simulink model "clutch_lockup"  (R2020a)
settings: Solver=VariableStepAuto  StartTime=0.0  StopTime=10.0  RelTol=1e-3
undefined symbols (not defined in the file or in its folder): be, bv, Ie, Iv, muk, mus, R
settings Model: Creator=Shubham  LastModifiedBy=Shubham

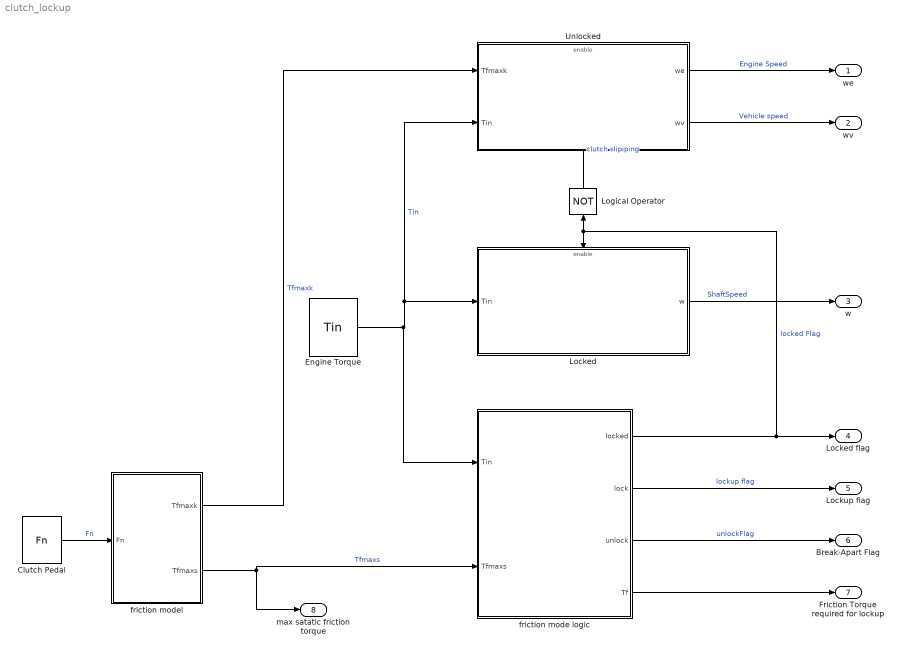
== system clutch_lockup ==
  Clutch Pedal : FromWorkspace  VariableName=Fn  ZeroCross=off
  Engine Torque : FromWorkspace  VariableName=Tin  ZeroCross=off
  Locked : Subsystem
  Logical Operator : Logic  Operator=NOT  IconShape=distinctive  AllPortsSameDT=off  OutDataTypeStr=boolean
  Unlocked : Subsystem
  friction mode logic : Subsystem  TreatAsAtomicUnit=on
  friction model : Subsystem
  we : Outport
  wv : Outport  Port=2
  w : Outport  Port=3
  Locked flag : Outport  Port=4
  Lockup flag : Outport  Port=5
  Break-Apart Flag : Outport  Port=6
  Friction Torque required for lockup : Outport  Port=7
  max satatic friction torque : Outport  Port=8
  wires:
  Engine Torque/1 -> friction mode logic/1(Tin), Locked/1(Tin), Unlocked/2(Tin)  "Tin"
  friction model/1(Tfmaxk) -> Unlocked/1(Tfmaxk)  "Tfmaxk"
  friction model/2(Tfmaxs) -> max satatic friction torque/1, friction mode logic/2(Tfmaxs)  "Tfmaxs"
  Clutch Pedal/1 -> friction model/1(Fn)  "Fn"
  Logical Operator/1 -> Unlocked/Enable  "clutch slipiping"
  Unlocked/1(we) -> we/1  "Engine Speed"
  Unlocked/2(wv) -> wv/1  "Vehicle speed"
  Locked/1(w) -> w/1  "ShaftSpeed"
  friction mode logic/2(lock) -> Lockup flag/1  "lockup flag"
  friction mode logic/3(unlock) -> Break-Apart Flag/1  "unlockFlag"
  friction mode logic/4(Tf) -> Friction Torque required for lockup/1
  friction mode logic/1(locked) -> Logical Operator/1, Locked/Enable, Locked flag/1  "locked Flag"

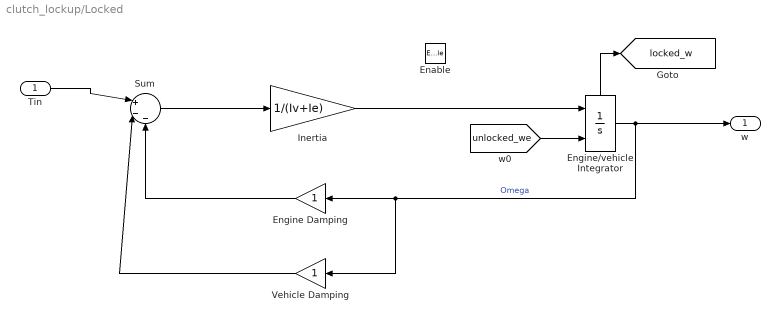
== system clutch_lockup/Locked ==
  Tin : Inport
  Enable : EnablePort  StatesWhenEnabling=reset
  Engine Damping : Gain
  Engine/vehicle Integrator : Integrator  InitialConditionSource=external  ShowStatePort=on
  Inertia : Gain  Gain=1/(Iv+Ie)
  Sum : Sum  Inputs=|+--
  Vehicle Damping : Gain
  w : Outport
  tag scope: locked_w=global
  wires:
  Sum/1 -> Inertia/1
  Inertia/1 -> Engine/vehicle Integrator/1
  Tin/1 -> Sum/1
  Engine/vehicle Integrator/State -> [locked_w]
  [unlocked_we] -> Engine/vehicle Integrator/2
  Engine Damping/1 -> Sum/3
  Vehicle Damping/1 -> Sum/2
  Engine/vehicle Integrator/1 -> w/1, Vehicle Damping/1, Engine Damping/1  "Omega"

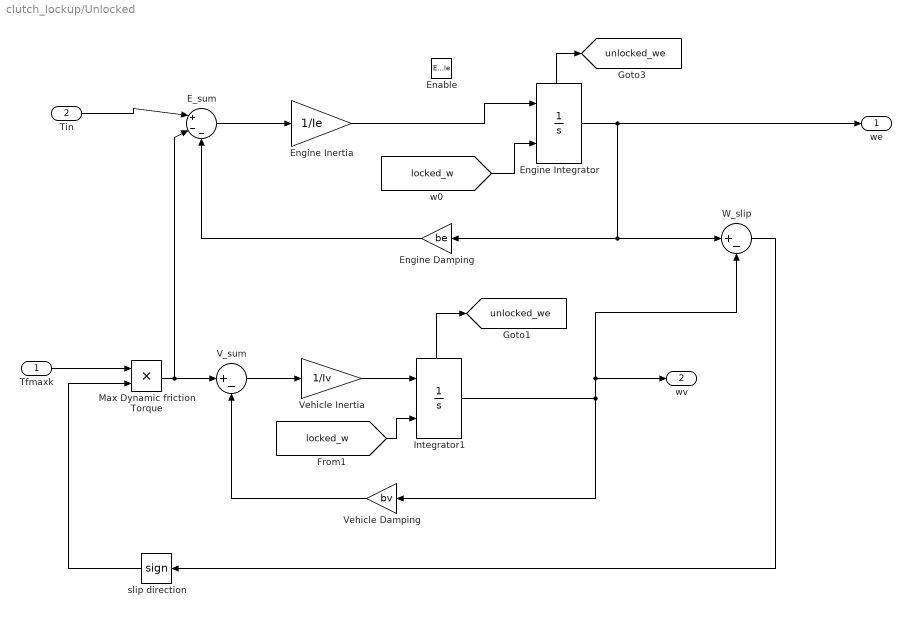
== system clutch_lockup/Unlocked ==
  Tfmaxk : Inport
  Tin : Inport  Port=2
  Enable : EnablePort  StatesWhenEnabling=reset
  E_sum : Sum  Inputs=|+--
  Engine Damping : Gain  Gain=be
  Engine Inertia : Gain  Gain=1/Ie
  Engine Integrator : Integrator  InitialConditionSource=external  ShowStatePort=on
  Integrator1 : Integrator  InitialConditionSource=external  ShowStatePort=on
  Max Dynamic friction Torque : Product
  V_sum : Sum  Inputs=|+-
  Vehicle Damping : Gain  Gain=bv
  Vehicle Inertia : Gain  Gain=1/Iv
  W_slip : Sum  Inputs=|+-
  slip direction : Signum
  we : Outport
  wv : Outport  Port=2
  tag scope: unlocked_we=global
  wires:
  Tin/1 -> E_sum/1
  E_sum/1 -> Engine Inertia/1
  Engine Inertia/1 -> Engine Integrator/1
  Engine Integrator/1 -> W_slip/1, Engine Damping/1, we/1
  Engine Damping/1 -> E_sum/3
  Vehicle Inertia/1 -> Integrator1/1
  V_sum/1 -> Vehicle Inertia/1
  Integrator1/1 -> W_slip/2, wv/1, Vehicle Damping/1
  Vehicle Damping/1 -> V_sum/2
  W_slip/1 -> slip direction/1
  slip direction/1 -> Max Dynamic friction Torque/2
  Max Dynamic friction Torque/1 -> E_sum/2, V_sum/1
  Tfmaxk/1 -> Max Dynamic friction Torque/1
  Engine Integrator/State -> [unlocked_we]
  Integrator1/State -> [unlocked_we]
  [locked_w] -> Engine Integrator/2
  [locked_w] -> Integrator1/2

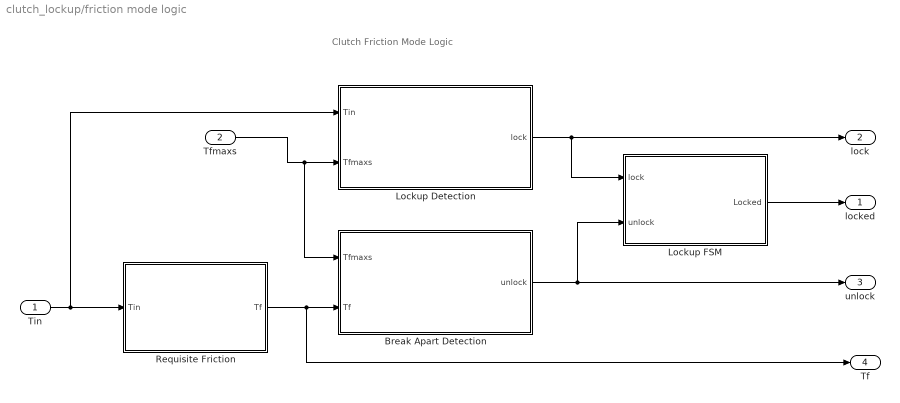
== system clutch_lockup/friction mode logic ==
  note: Clutch Friction Mode Logic
  Tin : Inport
  Tfmaxs : Inport  Port=2
  "Break Apart Detection " : Subsystem
  Lockup Detection : Subsystem
  Lockup FSM : Subsystem
  "Requisite Friction " : Subsystem
  locked : Outport
  lock : Outport  Port=2
  unlock : Outport  Port=3
  Tf : Outport  Port=4
  wires:
  "Requisite Friction "/1(Tf) -> "Break Apart Detection "/2(Tf), Tf/1
  Tin/1 -> "Requisite Friction "/1(Tin), Lockup Detection/1(Tin)
  Tfmaxs/1 -> "Break Apart Detection "/1(Tfmaxs), Lockup Detection/2(Tfmaxs)
  Lockup Detection/1(lock) -> Lockup FSM/1(lock), lock/1
  Lockup FSM/1(Locked) -> locked/1
  "Break Apart Detection "/1(unlock) -> Lockup FSM/2(unlock), unlock/1

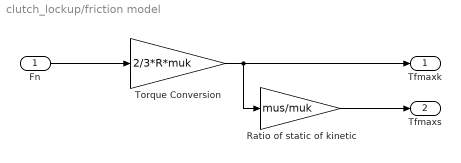
== system clutch_lockup/friction model ==
  Fn : Inport
  Ratio of static of kinetic : Gain  Gain=mus/muk
  Torque Conversion : Gain  Gain=2/3*R*muk
  Tfmaxk : Outport
  Tfmaxs : Outport  Port=2
  wires:
  Fn/1 -> Torque Conversion/1
  Torque Conversion/1 -> Tfmaxk/1, Ratio of static of kinetic/1
  Ratio of static of kinetic/1 -> Tfmaxs/1

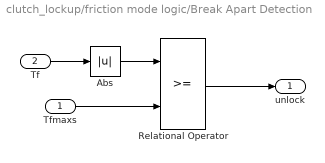
== system clutch_lockup/friction mode logic/Break Apart Detection  ==
  Tfmaxs : Inport
  Tf : Inport  Port=2
  Abs : Abs
  Relational Operator : RelationalOperator  OutDataTypeStr=boolean  RndMeth=Simplest
  unlock : Outport
  wires:
  Tf/1 -> Abs/1
  Relational Operator/1 -> unlock/1
  Abs/1 -> Relational Operator/1
  Tfmaxs/1 -> Relational Operator/2

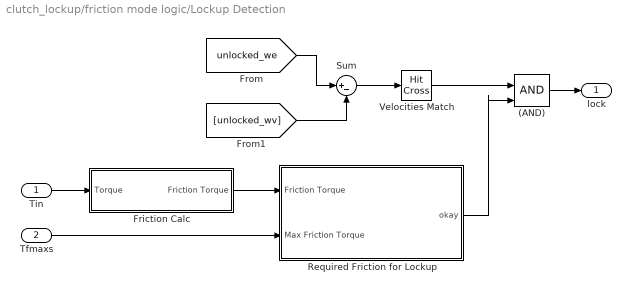
== system clutch_lockup/friction mode logic/Lockup Detection ==
  Tin : Inport
  Tfmaxs : Inport  Port=2
  (AND) : Logic  IconShape=distinctive  AllPortsSameDT=off  OutDataTypeStr=boolean
  Friction Calc : Subsystem
  Required Friction for Lockup : Subsystem
  Sum : Sum  Inputs=|+-
  Velocities Match : HitCross
  lock : Outport
  wires:
  Required Friction for Lockup/1(okay) -> (AND)/2
  (AND)/1 -> lock/1
  Tin/1 -> Friction Calc/1(Torque)
  Friction Calc/1(Friction Torque) -> Required Friction for Lockup/1(Friction Torque)
  Tfmaxs/1 -> Required Friction for Lockup/2(Max Friction Torque)
  Velocities Match/1 -> (AND)/1
  Sum/1 -> Velocities Match/1
  [unlocked_wv] -> Sum/2
  [unlocked_we] -> Sum/1

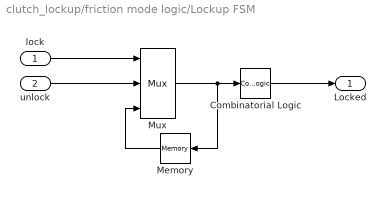
== system clutch_lockup/friction mode logic/Lockup FSM ==
  lock : Inport
  unlock : Inport  Port=2
  Combinatorial Logic : CombinatorialLogic  TruthTable=[0;1;0;0;1;1;1;0]
  Memory : Memory
  Mux : Mux  Inputs=3
  Locked : Outport
  wires:
  lock/1 -> Mux/1
  unlock/1 -> Mux/2
  Memory/1 -> Mux/3
  Mux/1 -> Memory/1, Combinatorial Logic/1
  Combinatorial Logic/1 -> Locked/1

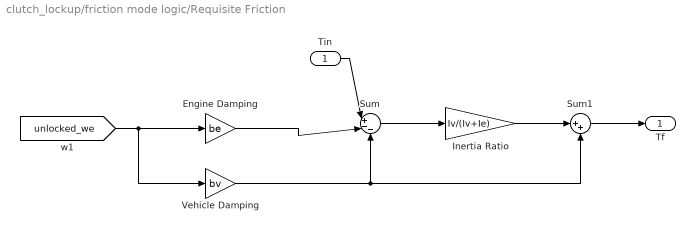
== system clutch_lockup/friction mode logic/Requisite Friction  ==
  Tin : Inport
  Engine Damping : Gain  Gain=be
  Inertia Ratio : Gain  Gain=Iv/(Iv+Ie)
  Sum : Sum  Inputs=|+--
  Sum1 : Sum  Inputs=|++
  Vehicle Damping : Gain  Gain=bv
  Tf : Outport
  wires:
  [unlocked_we] -> Vehicle Damping/1, Engine Damping/1
  Vehicle Damping/1 -> Sum1/2, Sum/3
  Sum1/1 -> Tf/1
  Tin/1 -> Sum/1
  Engine Damping/1 -> Sum/2
  Sum/1 -> Inertia Ratio/1
  Inertia Ratio/1 -> Sum1/1

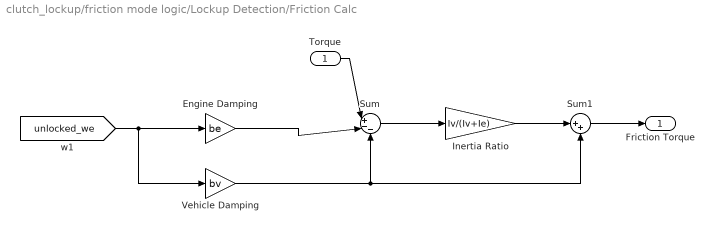
== system clutch_lockup/friction mode logic/Lockup Detection/Friction Calc ==
  Torque : Inport
  Engine Damping : Gain  Gain=be
  Inertia Ratio : Gain  Gain=Iv/(Iv+Ie)
  Sum : Sum  Inputs=|+--
  Sum1 : Sum  Inputs=|++
  Vehicle Damping : Gain  Gain=bv
  Friction Torque : Outport
  wires:
  [unlocked_we] -> Vehicle Damping/1, Engine Damping/1
  Torque/1 -> Sum/1
  Engine Damping/1 -> Sum/2
  Vehicle Damping/1 -> Sum1/2, Sum/3
  Sum/1 -> Inertia Ratio/1
  Inertia Ratio/1 -> Sum1/1
  Sum1/1 -> Friction Torque/1

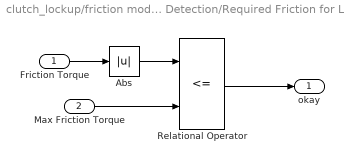
== system clutch_lockup/friction mode logic/Lockup Detection/Required Friction for Lockup ==
  Friction Torque : Inport
  Max Friction Torque : Inport  Port=2
  Abs : Abs
  Relational Operator : RelationalOperator  Operator=<=  OutDataTypeStr=boolean  RndMeth=Simplest
  okay : Outport
  wires:
  Relational Operator/1 -> okay/1
  Max Friction Torque/1 -> Relational Operator/2
  Friction Torque/1 -> Abs/1
  Abs/1 -> Relational Operator/1
